simulink model "Tut_8_StateLinearization_Backstepping"  (R2019b)
settings: Solver=FixedStepAuto  StartTime=0.0  StopTime=10.0  FixedStep=0.01  RelTol=1e-3
settings Model: Creator=김태욱  LastModifiedBy=김태욱

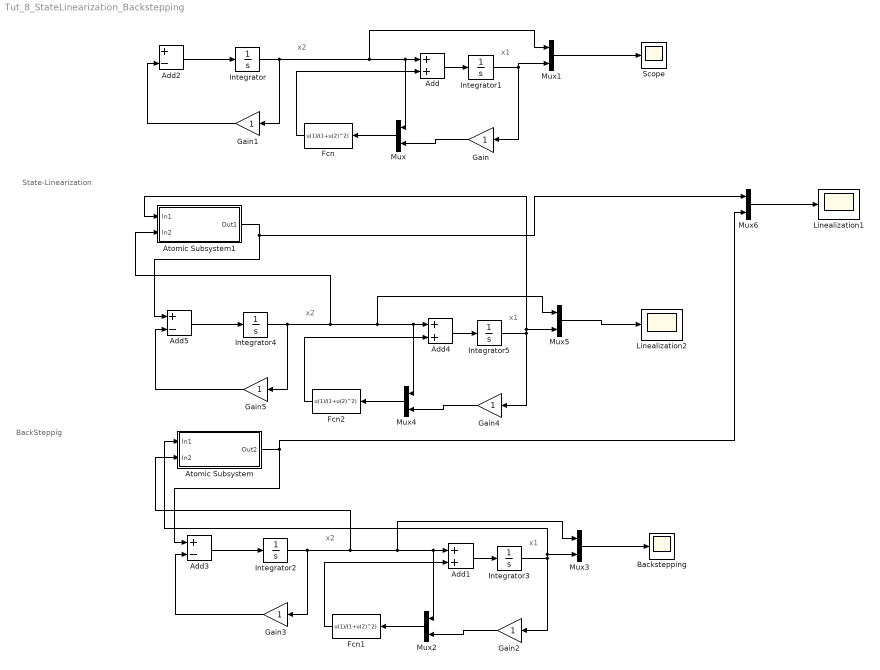
== system Tut_8_StateLinearization_Backstepping ==
  note: BackSteppig
  note: State-Linearization
  note: x2
  note: x1
  note: x2
  note: x1
  note: x2
  note: x1
  Add : Sum
  Add1 : Sum
  Add2 : Sum  Inputs=+-
  Add3 : Sum  Inputs=+-
  Add4 : Sum
  Add5 : Sum  Inputs=+-
  Atomic Subsystem : Subsystem  TreatAsAtomicUnit=on
  Atomic Subsystem1 : Subsystem  TreatAsAtomicUnit=on
  Backstepping : Scope
  Fcn : Fcn  Expr=u(1)/(1+u(2)^2)
  Fcn1 : Fcn  Expr=u(1)/(1+u(2)^2)
  Fcn2 : Fcn  Expr=u(1)/(1+u(2)^2)
  Gain{,1..5} (6 alike) : Gain
  Integrator{,1..5} (6 alike) : Integrator  InitialCondition=1
  Linealization1 : Scope
  Linealization2 : Scope
  Mux{,1..6} (7 alike) : Mux  Inputs=2
  Scope : Scope
  wires:
  Mux/1 -> Fcn/1
  Fcn/1 -> Add/2
  Integrator1/1 -> Gain/1, Mux1/2
  Integrator/1 -> Gain1/1, Mux1/1, Mux/1, Add/1
  Add/1 -> Integrator1/1
  Add2/1 -> Integrator/1
  Gain/1 -> Mux/2
  Mux1/1 -> Scope/1
  Gain1/1 -> Add2/2
  Add1/1 -> Integrator3/1
  Add3/1 -> Integrator2/1
  Gain3/1 -> Add3/2
  Gain2/1 -> Mux2/2
  Mux2/1 -> Fcn1/1
  Fcn1/1 -> Add1/2
  Mux3/1 -> Backstepping/1
  Integrator2/1 -> Atomic Subsystem/2(In2), Add1/1, Mux2/1, Mux3/1, Gain3/1
  Integrator3/1 -> Atomic Subsystem/1(In1), Mux3/2, Gain2/1
  Integrator4/1 -> Gain5/1, Mux5/1, Mux4/1, Add4/1, Atomic Subsystem1/2(In2)
  Add4/1 -> Integrator5/1
  Add5/1 -> Integrator4/1
  Fcn2/1 -> Add4/2
  Gain5/1 -> Add5/2
  Gain4/1 -> Mux4/2
  Mux4/1 -> Fcn2/1
  Integrator5/1 -> Gain4/1, Mux5/2, Atomic Subsystem1/1(In1)
  Mux5/1 -> Linealization2/1
  Atomic Subsystem/1(Out2) -> Add3/1, Mux6/2
  Mux6/1 -> Linealization1/1
  Atomic Subsystem1/1(Out1) -> Mux6/1, Add5/1

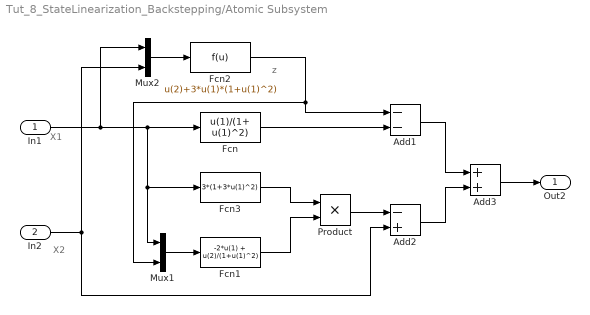
== system Tut_8_StateLinearization_Backstepping/Atomic Subsystem ==
  note: z
  note: X1
  note: X2
  In1 : Inport
  In2 : Inport  Port=2
  Add1 : Sum  Inputs=--
  Add2 : Sum  Inputs=-+
  Add3 : Sum
  Fcn : Fcn  Expr=u(1)/(1+ u(1)^2)
  Fcn1 : Fcn  Expr=-2*u(1) + u(2)/(1+u(1)^2)
  Fcn2 : Fcn  Expr=u(2)+3*u(1)*(1+u(1)^2)
  Fcn3 : Fcn  Expr=3*(1+3*u(1)^2)
  Mux1 : Mux  Inputs=2
  Mux2 : Mux  Inputs=2
  Product : Product
  Out2 : Outport
  wires:
  In1/1 -> Fcn3/1, Mux1/1, Fcn/1, Mux2/1
  In2/1 -> Add2/2, Mux2/2
  Mux2/1 -> Fcn2/1
  Mux1/1 -> Fcn1/1
  Fcn2/1 -> Add1/1, Mux1/2
  Fcn3/1 -> Product/1
  Fcn1/1 -> Product/2
  Fcn/1 -> Add1/2
  Product/1 -> Add2/1
  Add1/1 -> Add3/1
  Add2/1 -> Add3/2
  Add3/1 -> Out2/1

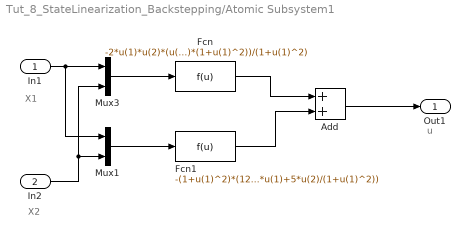
== system Tut_8_StateLinearization_Backstepping/Atomic Subsystem1 ==
  note: u
  note: X2
  note: X1
  In1 : Inport
  In2 : Inport  Port=2
  Add : Sum
  Fcn : Fcn  Expr=-2*u(1)*u(2)*(u(1)+u(2)*(1+u(1)^2))/(1+u(1)^2)
  Fcn1 : Fcn  Expr=-(1+u(1)^2)*(12*u(1)+5*u(2)/(1+u(1)^2))
  Mux1 : Mux  Inputs=2
  Mux3 : Mux  Inputs=2
  Out1 : Outport
  wires:
  In1/1 -> Mux1/1, Mux3/1
  In2/1 -> Mux1/2, Mux3/2
  Mux3/1 -> Fcn/1
  Mux1/1 -> Fcn1/1
  Fcn/1 -> Add/1
  Fcn1/1 -> Add/2
  Add/1 -> Out1/1
